simulink model "ysw5_8"  (R2014a)
settings: Solver=ode45  StartTime=0.0  StopTime=10.0  RelTol=1e-3
settings Model: Creator=Administrator  LastModifiedBy=Administrator

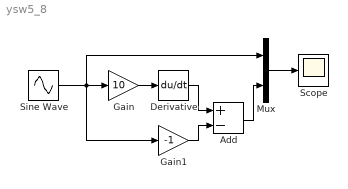
== system ysw5_8 ==
  Add : Sum  Inputs=+-
  Derivative : Derivative
  Gain : Gain  Gain=10
  Gain1 : Gain  Gain=-1
  Mux : Mux  Inputs=2
  Scope : Scope
  Sine Wave : Sin  SampleTime=0
  wires:
  Sine Wave/1 -> Gain1/1, Gain/1, Mux/1
  Mux/1 -> Scope/1
  Gain/1 -> Derivative/1
  Derivative/1 -> Add/1
  Gain1/1 -> Add/2
  Add/1 -> Mux/2
